simulink model "CTRL_TRGT_SADES_test"  (R2023b)
settings: Solver=VariableStepAuto  StartTime=0.0  StopTime=10.0  RelTol=1e-3
libraries: CTRL_TRGT_SADES x1
settings Model: Creator=blatak  LastModifiedBy=blatak

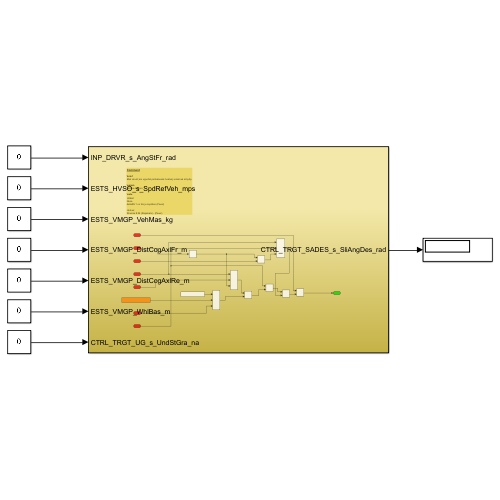
[thumbnail: Simulink's stored preview of the top-level diagram]
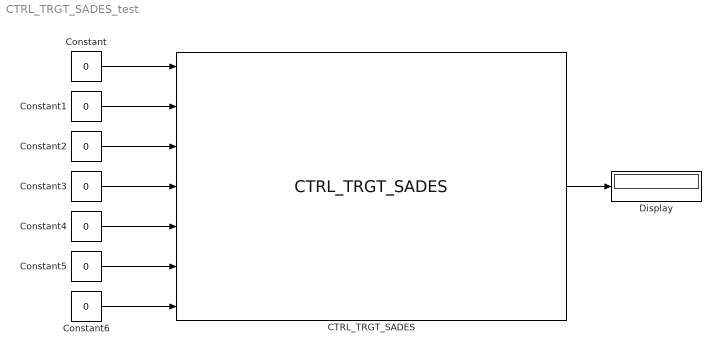
== system CTRL_TRGT_SADES_test ==
  CTRL_TRGT_SADES : CTRL_TRGT_SADES/CTRL_TRGT_SADES  SystemSampleTime=-1  VariantActivationTime=update diagram  AllowFlexibleInterface=on  Latency=0  AutoFrameSizeCalculation=off
  Constant{,1..6} (7 alike) : Constant  Value=0  OutDataTypeStr=single
  Display : Display
  wires:
  Constant/1 -> CTRL_TRGT_SADES/1
  Constant1/1 -> CTRL_TRGT_SADES/2
  Constant2/1 -> CTRL_TRGT_SADES/3
  Constant3/1 -> CTRL_TRGT_SADES/4
  Constant4/1 -> CTRL_TRGT_SADES/5
  Constant5/1 -> CTRL_TRGT_SADES/6
  Constant6/1 -> CTRL_TRGT_SADES/7
  CTRL_TRGT_SADES/1 -> Display/1
